simulink model "Terminal"  (R2018b)
settings: Solver=VariableStepAuto  StartTime=0.0  StopTime=100.0  RelTol=1e-3
undefined symbols (not defined in the file or in its folder): m, n
settings Model: Creator=Jorrit de Jong  LastModifiedBy=Jorrit de Jong

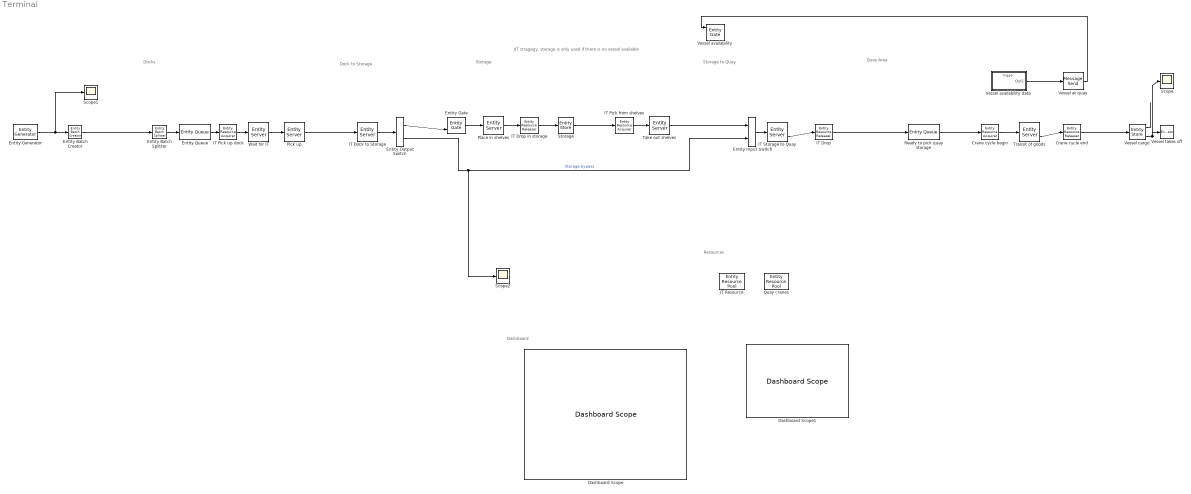
== system Terminal ==
  note: Dashboard
  note: JIT stragegy, storage is only used if there is no vessel available
  note: Docks
  note: Resources
  note: Storage
  note: Storage to Quay
  note: Quey Area
  note: Dock to Storage
  Crane cycle begin : EntityResourceAcquirer  InputPortMessageModes=m  OutputPortMessageModes=m  ResourceName=Crane
      settings: OutputPortMap=o3
  Crane cycle end : EntityResourceReleaser  InputPortMessageModes=m  OutputPortMessageModes=m  ResourceToRelease=Selected  ResourceName=Crane
  Dashboard Scope : DashboardScope  WebBlockId=48
  Dashboard Scope1 : DashboardScope  WebBlockId=52
  Entity Input Switch : EntityInputSwitch  InputPortMessageModes=m,m  OutputPortMessageModes=m
  Entity Output Switch : EntityOutputSwitch  InputPortMessageModes=m  OutputPortMessageModes=m,m  SwitchAttributeName=Attribute1  InitialPortSelection=2
  Entity Batch Creator : EntityBatchCreator  InputPortMessageModes=m  OutputPortMessageModes=m  NumberOfEntitiesInBatch=6
      settings: OutputPortMap=o4
  Entity Batch Splitter : EntityBatchSplitter  InputPortMessageModes=m  OutputPortMessageModes=m
      settings: OutputPortMap=o4
  Entity Gate : EntityGate  InputPortMessageModes=m,m  OutputPortMessageModes=m
  Entity Generator : EntityGenerator  OutputPortMessageModes=m  TimeSource=MATLAB action  IntergenerationTimeAction=|  EntityType=Structured  EntityTypeName=Entity
      | mu = 3;
      | sigma = 2;
      | dt = abs(normrnd(mu,sigma));
  Entity Queue : EntityQueue  InputPortMessageModes=m  OutputPortMessageModes=m
      settings: OutputPortMap=o5
  IT Dock to Storage : EntityServer  InputPortMessageModes=m  OutputPortMessageModes=m  Capacity=1
  IT Drop : EntityResourceReleaser  InputPortMessageModes=m  OutputPortMessageModes=m  ResourceToRelease=Selected  ResourceName=IT
  IT Drop in storage : EntityResourceReleaser  InputPortMessageModes=m  OutputPortMessageModes=m  ResourceToRelease=Selected  ResourceName=IT
  IT Pick from shelves : EntityResourceAcquirer  InputPortMessageModes=m  OutputPortMessageModes=m  ResourceName=IT
      settings: OutputPortMap=o3
  IT Pick up dock : EntityResourceAcquirer  InputPortMessageModes=m  OutputPortMessageModes=m  ResourceName=IT
      settings: OutputPortMap=o3
  IT Resource : EntityResourcePool  ResourceName=IT  ResourceAmount=5
  IT Storage to Quay : EntityServer  InputPortMessageModes=m  OutputPortMessageModes=n,m  Capacity=1  NumberEntitiesDeparted=on
      settings: OutputPortMap=o0,o9
  Pick up : EntityServer  InputPortMessageModes=m  OutputPortMessageModes=m  Capacity=1
  Place in shelves : EntityServer  InputPortMessageModes=m  OutputPortMessageModes=m  Capacity=1
  Quay cranes : EntityResourcePool  ResourceName=Crane  ResourceAmount=2
  Ready to pick quay storage : EntityQueue  InputPortMessageModes=m  OutputPortMessageModes=m
      settings: OutputPortMap=o5
  Scope : Scope
  Scope1 : Scope
  Scope2 : Scope
  Storage : EntityStore  InputPortMessageModes=m  OutputPortMessageModes=m
      settings: OutputPortMap=o4
  Take out shelves : EntityServer  InputPortMessageModes=m  OutputPortMessageModes=m  Capacity=1
  Transit of goods : EntityServer  InputPortMessageModes=m  OutputPortMessageModes=n,m  Capacity=inf  ServiceTimeSource=MATLAB action  ServiceTimeValue=30  ServiceTimeAction=|  NumberEntitiesDeparted=on
      | mu = 30;
      | sigma = 5;
      | dt = abs(normrnd(mu,sigma));
      settings: OutputPortMap=o0,o9
  Vessel at quay : MessageSend  OutputPortMessageModes=m
      settings: InputPortMap=u1
  Vessel availability : EntityGate  InputPortMessageModes=m,m  OutputPortMessageModes=m
  Vessel availability data : Subsystem  TreatAsAtomicUnit=on
  Vessel cargo : EntityStore  InputPortMessageModes=m  OutputPortMessageModes=n,m  NumberEntitiesDeparted=on
      settings: OutputPortMap=o0,o4
  Vessel takes off : EntityTerminator  InputPortMessageModes=m  NumberEntitiesArrived=on
      settings: OutputPortMap=o0
  Wait for IT : EntityServer  InputPortMessageModes=m  OutputPortMessageModes=m  Capacity=1
  wires:
  Vessel cargo/2 -> Scope/1, Vessel takes off/1
  Crane cycle end/1 -> Vessel cargo/1
  Crane cycle begin/1 -> Transit of goods/1
  Transit of goods/2 -> Crane cycle end/1
  Vessel at quay/1 -> Vessel availability/1
  Vessel availability data/1(Out1) -> Vessel at quay/1
  IT Storage to Quay/2 -> IT Drop/1
  Ready to pick quay storage/1 -> Crane cycle begin/1
  IT Drop/1 -> Ready to pick quay storage/1
  IT Dock to Storage/1 -> Entity Output Switch/1
  Wait for IT/1 -> Pick up/1
  Entity Batch Creator/1 -> Entity Batch Splitter/1
  Entity Input Switch/1 -> IT Storage to Quay/1
  IT Pick from shelves/1 -> Take out shelves/1
  Entity Output Switch/2 -> Scope2/1, Entity Input Switch/2  "Storage bypass"
  Take out shelves/1 -> Entity Input Switch/1
  Place in shelves/1 -> IT Drop in storage/1
  IT Drop in storage/1 -> Storage/1
  Entity Queue/1 -> IT Pick up dock/1
  IT Pick up dock/1 -> Wait for IT/1
  Entity Batch Splitter/1 -> Entity Queue/1
  Pick up/1 -> IT Dock to Storage/1
  Entity Generator/1 -> Scope1/1, Entity Batch Creator/1
  Entity Output Switch/1 -> Entity Gate/2
  Entity Gate/1 -> Place in shelves/1
  Storage/1 -> IT Pick from shelves/1
  Vessel cargo/1 -> ?

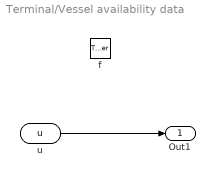
== system Terminal/Vessel availability data ==
  f : TriggerPort  TriggerType=function-call  IsSimulinkFunction=on  FunctionName=f  FunctionVisibility=scoped  VariantControl=(inherit)
  u : ArgIn  DisableCoverage=on  ArgumentName=u
  Out1 : Outport
  wires:
  u/1 -> Out1/1
